simulink model "Model_3b"  (R2020b)
settings: Solver=VariableStepAuto  StartTime=0.0  StopTime=10.0  RelTol=1e-3
settings Model: Creator=Akarsh  LastModifiedBy=Akarsh

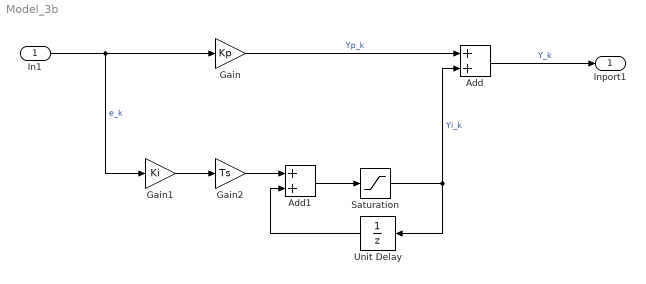
== system Model_3b ==
  In1 : Inport  OutDataTypeStr=double  PortDimensions=1  SampleTime=0
  Add : Sum
  Add1 : Sum
  Gain : Gain  Gain=Kp  mask{Kp=336, Parameter2=200}
  Gain1 : Gain  Gain=Ki  mask{Ki=44}
  Gain2 : Gain  Gain=Ts  mask{Ts=0.01}
  Saturation : Saturate  UpperLimit=1  LowerLimit=-1
  Unit Delay : UnitDelay  SampleTime=-1  HasFrameUpgradeWarning=on
  Inport1 : Outport  OutDataTypeStr=double  PortDimensions=1  SampleTime=0
  wires:
  Gain2/1 -> Add1/1
  Gain1/1 -> Gain2/1
  Gain/1 -> Add/1  "Yp_k"
  Saturation/1 -> Unit Delay/1, Add/2  "Yi_k"
  Add/1 -> Inport1/1  "Y_k"
  Add1/1 -> Saturation/1
  Unit Delay/1 -> Add1/2
  In1/1 -> Gain/1, Gain1/1  "e_k"
